simulink model "simulink_both_machines"  (R2020b)
settings: Solver=FixedStepDiscrete  StartTime=0.0  StopTime=10.0  FixedStep=5000  RelTol=1e-3
settings Model: Creator=Ahmed Zaghloul  LastModifiedBy=Ahmed Zaghloul

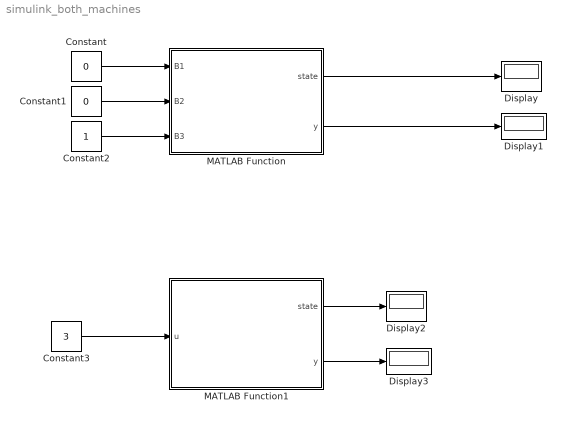
== system simulink_both_machines ==
  Constant : Constant  Value=0
  Constant1 : Constant  Value=0
  Constant2 : Constant
  Constant3 : Constant  Value=3
  Display{,1..3} (4 alike) : Display
  MATLAB Function : MATLAB Function  TreatAsAtomicUnit=on
  MATLAB Function1 : MATLAB Function  TreatAsAtomicUnit=on
  wires:
  MATLAB Function/1(state) -> Display/1
  MATLAB Function/2(y) -> Display1/1
  Constant/1 -> MATLAB Function/1(B1)
  Constant1/1 -> MATLAB Function/2(B2)
  Constant2/1 -> MATLAB Function/3(B3)
  Constant3/1 -> MATLAB Function1/1(u)
  MATLAB Function1/1(state) -> Display2/1
  MATLAB Function1/2(y) -> Display3/1

== matlab function simulink_both_machines/MATLAB Function1 ==
  data: state output; u input; y output
function [state ,y] = fcn(u)
persistent current_state
if(isempty(current_state))
    current_state = 1;
end
switch current_state
    case 1
        switch u
            case 1
                current_state = 1;
            case 2
                current_state = 4;
            otherwise
                current_state = 6;
        end
    case 2
        switch u
            case 1
                current_state = 5;
            case 2
                current_state = 2;
            otherwise
                current_state = 8;
        end
    case 3
        switch u
            case 1
                current_state = 7;
            case 2
                current_state = 9;
            otherwise
                current_state = 3;
        end
    case 4
        switch u
            case 2
                current_state = 2;
        end
    case 5
        switch u
            case 1
                current_state = 1;
        end
    case 6
        switch u
            case 3
                current_state = 3;
        end  
    case 7
        switch u
            case 1
                current_state = 1;
        end  
    case 8
        switch u
            case 3
                current_state = 3;
        end  
    case 9
        switch u
            case 2
                current_state = 2;
        end  
end
switch current_state
    case 1
        y = "s";
    case 2
        y = "s";
    case 3
        y = "s";
    case 4
        y = "u1";
    case 5
        y = "u1";
    case 6
        y = "u2";
    case 7
        y = "d2";
    case 8
        y = "u1";
    otherwise
        y = "d1";
end
state = current_state;
end

== matlab function simulink_both_machines/MATLAB Function ==
  data: state output; B1 input; y output; B2 input; B3 input
function [state,y] = fcn(B1,B2,B3)
persistent current_state
if(isempty(current_state))
    current_state = 1;
end
switch current_state
    case 1
        if(B2)
            current_state = 2;
            y = "u1";
        elseif(B3)
            current_state = 3;
            y = "u2";
        else
            current_state = 1;
            y = "s";
        end
    case 2
        if(B1)
            current_state = 1;
            y = "d1";
        elseif(B3)
            current_state = 3;
            y = "u1";
        else
            current_state = 2;
            y = "s";
        end
    otherwise
        if(B1)
            current_state = 1;
            y = "d2";
        elseif(B2)
            current_state = 2;
            y = "d1";
        else
            current_state = 3;
            y = "s";
        end
end
state = current_state;
end
